simulink model "vending_machine"  (R2020b)
settings: Solver=VariableStepAuto  StartTime=0.0  StopTime=10.0  RelTol=1e-3
settings Model: Creator=Varun  LastModifiedBy=Varun

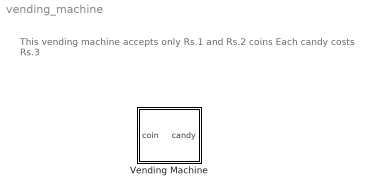
== system vending_machine ==
  note: This vending machine accepts only Rs.1 and Rs.2 coins
      | Each candy costs Rs.3
  Vending Machine : Stateflow chart  TreatAsAtomicUnit=on

== stateflow chart vending_machine/Vending Machine ==
  state Got_Rs_2
  state Got_none
  state Got_Rs_1
  Got_Rs_2 -> Got_none [order 1] : [coin==1]{candy=1}
  Got_none -> Got_Rs_2 [order 2] : [coin==2]{candy=0}
  Got_Rs_1 -> Got_Rs_2 [order 2] : [coin==1]{candy=0}
  Got_Rs_2 -> Got_Rs_1 [order 2] : [coin==2]{candy=1}
  Got_Rs_1 -> Got_none [order 1] : [coin==2]{candy=1}
  (default) -> Got_none
  Got_none -> Got_Rs_1 [order 1] : [coin==1]{candy=0}
  data: coin input; candy output
